simulink subsystem "SelfDefined_Two_Level_Converter"  (R2024b)
settings: Solver=VariableStepAuto  StartTime=0.0  StopTime=10.0  RelTol=1e-3
libraries: spsIGBTDiodeLib x6, simulink x1
settings Model: Creator=XixiLab  LastModifiedBy=XixiLab

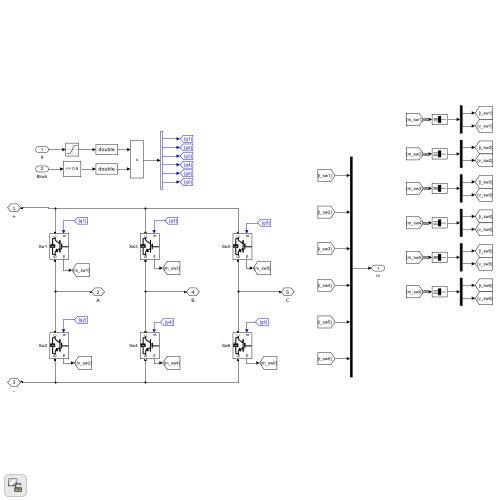
[thumbnail: Simulink's stored preview of the top-level diagram]
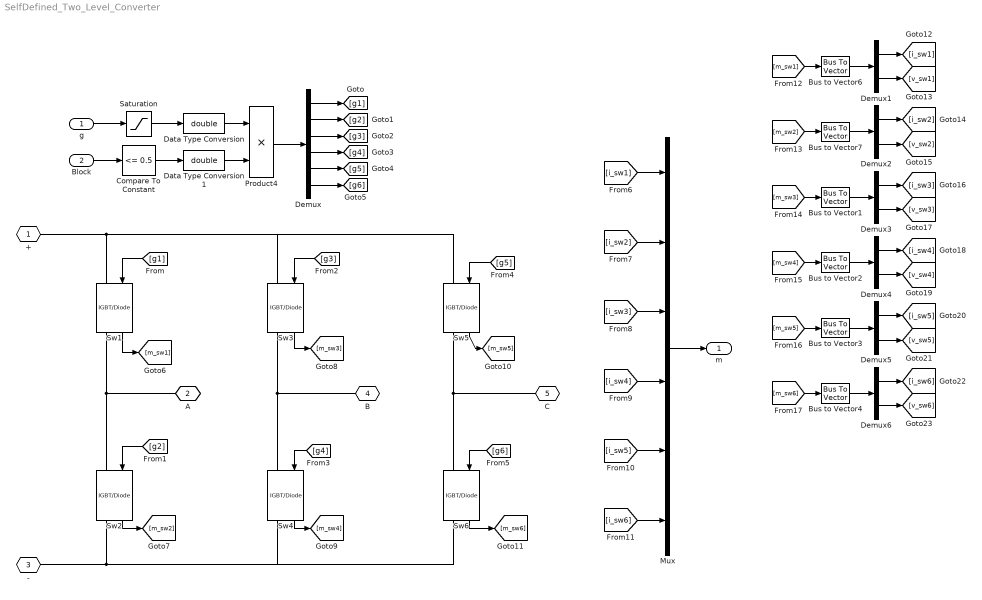
== system SelfDefined_Two_Level_Converter ==
  g : Inport  PortDimensions=6
  Block : Inport  Port=2  PortDimensions=1
  Bus to Vector{1..4,6..7} (6 alike) : BusToVector
  Compare To Constant : simulink/Logic and Bit Operations/Compare To Constant  relop=<=  const=0.5  OutDataTypeStr=boolean
  Data Type Conversion : DataTypeConversion  OutDataTypeStr=double  SaturateOnIntegerOverflow=off  RndMeth=Floor
  Data Type Conversion1 : DataTypeConversion  OutDataTypeStr=double  SaturateOnIntegerOverflow=off  RndMeth=Floor
  Demux : Demux  Outputs=6
  Demux{1..6} (6 alike) : Demux  Outputs=2
  Mux : Mux  Inputs=6
  Product4 : Product
  Saturation : Saturate  UpperLimit=1  LowerLimit=0
  Sw{1..6} (6 alike) : spsIGBTDiodeLib/IGBT//Diode  Ron=1e-3  Rs=1e6  Cs=inf  Measurements=on
  + : PMIOPort  Tag=PMCPort  Side=Right
  A : PMIOPort  Tag=PMCPort  Port=2  Side=Left
  - : PMIOPort  Tag=PMCPort  Port=3  Side=Right
  B : PMIOPort  Tag=PMCPort  Port=4  Side=Left
  C : PMIOPort  Tag=PMCPort  Port=5  Side=Left
  m : Outport
  wires:
  Demux/1 -> [g1]
  Block/1 -> Compare To Constant/1
  Demux/2 -> [g2]
  Demux/4 -> [g4]
  [g1] -> Sw1/1
  [g3] -> Sw3/1
  Demux/3 -> [g3]
  Data Type Conversion1/1 -> Product4/2
  [g6] -> Sw6/1
  Saturation/1 -> Data Type Conversion/1
  g/1 -> Saturation/1
  Demux/6 -> [g6]
  Data Type Conversion/1 -> Product4/1
  Compare To Constant/1 -> Data Type Conversion1/1
  [g4] -> Sw4/1
  Product4/1 -> Demux/1
  Demux/5 -> [g5]
  [g5] -> Sw5/1
  [g2] -> Sw2/1
  Mux/1 -> m/1
  Sw1/1 -> [m_sw1]
  Sw2/1 -> [m_sw2]
  Sw3/1 -> [m_sw3]
  Sw4/1 -> [m_sw4]
  Sw5/1 -> [m_sw5]
  Sw6/1 -> [m_sw6]
  [i_sw1] -> Mux/1
  [i_sw2] -> Mux/2
  [i_sw3] -> Mux/3
  [i_sw4] -> Mux/4
  [i_sw5] -> Mux/5
  [i_sw6] -> Mux/6
  [m_sw1] -> Bus to Vector6/1
  Bus to Vector6/1 -> Demux1/1
  Demux1/1 -> [i_sw1]
  Demux1/2 -> [v_sw1]
  Demux2/1 -> [i_sw2]
  Bus to Vector7/1 -> Demux2/1
  Demux2/2 -> [v_sw2]
  [m_sw2] -> Bus to Vector7/1
  [m_sw3] -> Bus to Vector1/1
  Bus to Vector1/1 -> Demux3/1
  Demux3/1 -> [i_sw3]
  Demux3/2 -> [v_sw3]
  Demux4/2 -> [v_sw4]
  Demux4/1 -> [i_sw4]
  [m_sw4] -> Bus to Vector2/1
  Bus to Vector2/1 -> Demux4/1
  Demux5/2 -> [v_sw5]
  Demux5/1 -> [i_sw5]
  [m_sw5] -> Bus to Vector3/1
  Bus to Vector3/1 -> Demux5/1
  Demux6/2 -> [v_sw6]
  Demux6/1 -> [i_sw6]
  [m_sw6] -> Bus to Vector4/1
  Bus to Vector4/1 -> Demux6/1
  connections:
  +/RConn1 -- Sw5/LConn1 -- Sw3/LConn1 -- Sw1/LConn1
  A/RConn1 -- Sw2/LConn1 -- Sw1/RConn1
  -/RConn1 -- Sw6/RConn1 -- Sw4/RConn1 -- Sw2/RConn1
  Sw4/LConn1 -- B/RConn1 -- Sw3/RConn1
  Sw5/RConn1 -- C/RConn1 -- Sw6/LConn1
